simulink model "atrias"  (R2014a)
settings: Solver=FixedStepDiscrete  StartTime=0.0  StopTime=inf  FixedStep=0.001  RelTol=1e-3
libraries: xpcethercatlib x57, simulink x8, slrtlib x7
settings Model: xpc_rtwmakecfg_data=_xpcethercatlib_  SimulationMode=external  BufferReuse=off  Creator=drl  LastModifiedBy=drl
settings SolverCC: EnableConcurrentExecution=on  ConcurrentTasks=on
settings OptimizationCC: BlockReduction=off  OptimizeBlockIOStorage=off  BufferReuse=off  GlobalBufferReuse=off  ExpressionFolding=off  LocalBlockOutputs=off
settings HardwareCC: ProdIntDivRoundTo=Zero  ProdEndianess=LittleEndian  ProdHWDeviceType=Generic->32-bit x86 compatible
settings RTWCC: SystemTargetFile=slrt.tlc  TemplateMakefile=slrt_default_tmf  Description=Simulink Real-Time  ProcessScript=slrt_make_rtw_hook  RTWCompilerOptimization=On
settings SimulinkRealTimeCC: GeneratePreprocessorConditionals=Disable all  EnableShiftOperators=on

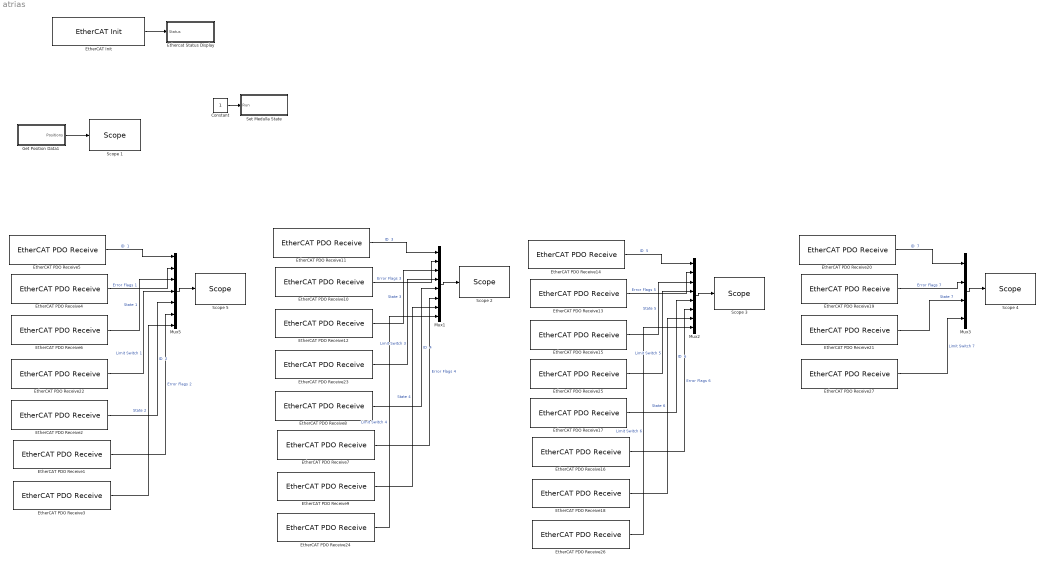
== system atrias ==
  Constant : Constant
  "EtherCAT Init " : xpcethercatlib/EtherCAT Init   Priority=0  config_file=C:\Users\drl\Documents\MATLAB\eni_atrias.xml  device_id=0  pci_bus=4  pci_slot=0  enaDebug=off  enaDC=on  errLink=off  masterDbg=off  stateChgDbg=off  baseClock=off  masterCfg=off  logFile='c:\dbglog.txt'  sample_time=0.001000
  EtherCAT PDO Receive1 : xpcethercatlib/EtherCAT PDO Receive  Priority=2  sig_name=Box 2 (ATRIAS 2.1 Boom (Medulla 1.5)).uController Status.Error Flags  sig_offset=992  sig_type=uint8  type_size=8  sig_dim=1  device_id=0  sample_time=0.001000
  EtherCAT PDO Receive10 : xpcethercatlib/EtherCAT PDO Receive  Priority=2  sig_name=Box 3 (ATRIAS 2.1 Hip (Medulla 1.5)).uController Status.Error Flags  sig_offset=1184  sig_type=uint8  type_size=8  sig_dim=1  device_id=0  sample_time=0.001000
  EtherCAT PDO Receive11 : xpcethercatlib/EtherCAT PDO Receive  Priority=2  sig_name=Box 3 (ATRIAS 2.1 Hip (Medulla 1.5)).uController Status.ID  sig_offset=1160  sig_type=uint8  type_size=8  sig_dim=1  device_id=0  sample_time=0.001000
  EtherCAT PDO Receive12 : xpcethercatlib/EtherCAT PDO Receive  Priority=2  sig_name=Box 3 (ATRIAS 2.1 Hip (Medulla 1.5)).uController Status.State  sig_offset=1168  sig_type=uint8  type_size=8  sig_dim=1  device_id=0  sample_time=0.001000
  EtherCAT PDO Receive13 : xpcethercatlib/EtherCAT PDO Receive  Priority=2  sig_name=Box 5 (ATRIAS 2.1 Leg (Medulla 1.5)).uController Status.Error Flags  sig_offset=1808  sig_type=uint8  type_size=8  sig_dim=1  device_id=0  sample_time=0.001000
  EtherCAT PDO Receive14 : xpcethercatlib/EtherCAT PDO Receive  Priority=2  sig_name=Box 5 (ATRIAS 2.1 Leg (Medulla 1.5)).uController Status.ID  sig_offset=1784  sig_type=uint8  type_size=8  sig_dim=1  device_id=0  sample_time=0.001000
  EtherCAT PDO Receive15 : xpcethercatlib/EtherCAT PDO Receive  Priority=2  sig_name=Box 5 (ATRIAS 2.1 Leg (Medulla 1.5)).uController Status.State  sig_offset=1792  sig_type=uint8  type_size=8  sig_dim=1  device_id=0  sample_time=0.001000
  EtherCAT PDO Receive16 : xpcethercatlib/EtherCAT PDO Receive  Priority=2  sig_name=Box 6 (ATRIAS 2.1 Leg (Medulla 1.5)).uController Status.Error Flags  sig_offset=2184  sig_type=uint8  type_size=8  sig_dim=1  device_id=0  sample_time=0.001000
  EtherCAT PDO Receive17 : xpcethercatlib/EtherCAT PDO Receive  Priority=2  sig_name=Box 6 (ATRIAS 2.1 Leg (Medulla 1.5)).uController Status.ID  sig_offset=2160  sig_type=uint8  type_size=8  sig_dim=1  device_id=0  sample_time=0.001000
  EtherCAT PDO Receive18 : xpcethercatlib/EtherCAT PDO Receive  Priority=2  sig_name=Box 6 (ATRIAS 2.1 Leg (Medulla 1.5)).uController Status.State  sig_offset=2168  sig_type=uint8  type_size=8  sig_dim=1  device_id=0  sample_time=0.001000
  EtherCAT PDO Receive19 : xpcethercatlib/EtherCAT PDO Receive  Priority=2  sig_name=Box 7 (ATRIAS 2.1 Hip (Medulla 1.5)).uController Status.Error Flags  sig_offset=2560  sig_type=uint8  type_size=8  sig_dim=1  device_id=0  sample_time=0.001000
  EtherCAT PDO Receive2 : xpcethercatlib/EtherCAT PDO Receive  Priority=2  sig_name=Box 2 (ATRIAS 2.1 Boom (Medulla 1.5)).uController Status.ID  sig_offset=968  sig_type=uint8  type_size=8  sig_dim=1  device_id=0  sample_time=0.001000
  EtherCAT PDO Receive20 : xpcethercatlib/EtherCAT PDO Receive  Priority=2  sig_name=Box 7 (ATRIAS 2.1 Hip (Medulla 1.5)).uController Status.ID  sig_offset=2536  sig_type=uint8  type_size=8  sig_dim=1  device_id=0  sample_time=0.001000
  EtherCAT PDO Receive21 : xpcethercatlib/EtherCAT PDO Receive  Priority=2  sig_name=Box 7 (ATRIAS 2.1 Hip (Medulla 1.5)).uController Status.State  sig_offset=2544  sig_type=uint8  type_size=8  sig_dim=1  device_id=0  sample_time=0.001000
  EtherCAT PDO Receive22 : xpcethercatlib/EtherCAT PDO Receive  Priority=2  sig_name=Box 1 (ATRIAS 2.1 Leg (Medulla 1.5)).uController Status.Limit Switch  sig_offset=624  sig_type=uint8  type_size=8  sig_dim=1  device_id=0  sample_time=0.001000
  EtherCAT PDO Receive23 : xpcethercatlib/EtherCAT PDO Receive  Priority=2  sig_name=Box 3 (ATRIAS 2.1 Hip (Medulla 1.5)).uController Status.Limit Switch  sig_offset=1192  sig_type=uint8  type_size=8  sig_dim=1  device_id=0  sample_time=0.001000
  EtherCAT PDO Receive24 : xpcethercatlib/EtherCAT PDO Receive  Priority=2  sig_name=Box 4 (ATRIAS 2.1 Leg (Medulla 1.5)).uController Status.Limit Switch  sig_offset=1440  sig_type=uint8  type_size=8  sig_dim=1  device_id=0  sample_time=0.001000
  EtherCAT PDO Receive25 : xpcethercatlib/EtherCAT PDO Receive  Priority=2  sig_name=Box 5 (ATRIAS 2.1 Leg (Medulla 1.5)).uController Status.Limit Switch  sig_offset=1816  sig_type=uint8  type_size=8  sig_dim=1  device_id=0  sample_time=0.001000
  EtherCAT PDO Receive26 : xpcethercatlib/EtherCAT PDO Receive  Priority=2  sig_name=Box 6 (ATRIAS 2.1 Leg (Medulla 1.5)).uController Status.State  sig_offset=2168  sig_type=uint8  type_size=8  sig_dim=1  device_id=0  sample_time=0.001000
  EtherCAT PDO Receive27 : xpcethercatlib/EtherCAT PDO Receive  Priority=2  sig_name=Box 7 (ATRIAS 2.1 Hip (Medulla 1.5)).uController Status.Limit Switch  sig_offset=2568  sig_type=uint8  type_size=8  sig_dim=1  device_id=0  sample_time=0.001000
  EtherCAT PDO Receive3 : xpcethercatlib/EtherCAT PDO Receive  Priority=2  sig_name=Box 2 (ATRIAS 2.1 Boom (Medulla 1.5)).uController Status.State  sig_offset=976  sig_type=uint8  type_size=8  sig_dim=1  device_id=0  sample_time=0.001000
  EtherCAT PDO Receive4 : xpcethercatlib/EtherCAT PDO Receive  Priority=2  sig_name=Box 1 (ATRIAS 2.1 Leg (Medulla 1.5)).uController Status.Error Flags  sig_offset=616  sig_type=uint8  type_size=8  sig_dim=1  device_id=0  sample_time=0.001000
  EtherCAT PDO Receive5 : xpcethercatlib/EtherCAT PDO Receive  Priority=2  sig_name=Box 1 (ATRIAS 2.1 Leg (Medulla 1.5)).uController Status.ID  sig_offset=592  sig_type=uint8  type_size=8  sig_dim=1  device_id=0  sample_time=0.001000
  EtherCAT PDO Receive6 : xpcethercatlib/EtherCAT PDO Receive  Priority=2  sig_name=Box 1 (ATRIAS 2.1 Leg (Medulla 1.5)).uController Status.State  sig_offset=600  sig_type=uint8  type_size=8  sig_dim=1  device_id=0  sample_time=0.001000
  EtherCAT PDO Receive7 : xpcethercatlib/EtherCAT PDO Receive  Priority=2  sig_name=Box 4 (ATRIAS 2.1 Leg (Medulla 1.5)).uController Status.Error Flags  sig_offset=1432  sig_type=uint8  type_size=8  sig_dim=1  device_id=0  sample_time=0.001000
  EtherCAT PDO Receive8 : xpcethercatlib/EtherCAT PDO Receive  Priority=2  sig_name=Box 4 (ATRIAS 2.1 Leg (Medulla 1.5)).uController Status.ID  sig_offset=1408  sig_type=uint8  type_size=8  sig_dim=1  device_id=0  sample_time=0.001000
  EtherCAT PDO Receive9 : xpcethercatlib/EtherCAT PDO Receive  Priority=2  sig_name=Box 4 (ATRIAS 2.1 Leg (Medulla 1.5)).uController Status.State  sig_offset=1416  sig_type=uint8  type_size=8  sig_dim=1  device_id=0  sample_time=0.001000
  Ethercat Status Display : Subsystem
  Get Position Data1 : Subsystem
  Mux1 : Mux  Inputs=8
  Mux2 : Mux  Inputs=8
  Mux3 : Mux
  Mux5 : Mux  Inputs=7
  Scope 1 : slrtlib/Displays and Logging/Scope   scopeno=1  scopetype=Target  autostart=on  viewmode=Numerical  formatstr='%15.6f'  grid=on  ylimits=[0,0]  nosamples=100  noprepostsamples=0  interleave=1  triggermode=FreeRun  triggersignal=1  trigsignalfromport=off  triggerlevel=0.0  triggerslope=Either  triggerscope=1  triggersample=0  filename=data.dat  mode=Lazy  writesize=512  autorestart=off  dynamicfilemode=off  maxwritefilesize=512*1024^2
  Scope 2 : slrtlib/Displays and Logging/Scope   scopeno=4  scopetype=Target  autostart=on  viewmode=Numerical  formatstr='%15.6f'  grid=on  ylimits=[0,0]  nosamples=100  noprepostsamples=0  interleave=1  triggermode=FreeRun  triggersignal=1  trigsignalfromport=off  triggerlevel=0.0  triggerslope=Either  triggerscope=1  triggersample=0  filename=data.dat  mode=Lazy  writesize=512  autorestart=off  dynamicfilemode=off  maxwritefilesize=512*1024^2
  Scope 3 : slrtlib/Displays and Logging/Scope   scopeno=5  scopetype=Target  autostart=on  viewmode=Numerical  formatstr='%15.6f'  grid=on  ylimits=[0,0]  nosamples=100  noprepostsamples=0  interleave=1  triggermode=FreeRun  triggersignal=1  trigsignalfromport=off  triggerlevel=0.0  triggerslope=Either  triggerscope=1  triggersample=0  filename=data.dat  mode=Lazy  writesize=512  autorestart=off  dynamicfilemode=off  maxwritefilesize=512*1024^2
  Scope 4 : slrtlib/Displays and Logging/Scope   scopeno=7  scopetype=Target  autostart=on  viewmode=Numerical  formatstr='%15.6f'  grid=on  ylimits=[0,0]  nosamples=100  noprepostsamples=0  interleave=1  triggermode=FreeRun  triggersignal=1  trigsignalfromport=off  triggerlevel=0.0  triggerslope=Either  triggerscope=1  triggersample=0  filename=data.dat  mode=Lazy  writesize=512  autorestart=off  dynamicfilemode=off  maxwritefilesize=512*1024^2
  Scope 5 : slrtlib/Displays and Logging/Scope   scopeno=3  scopetype=Target  autostart=on  viewmode=Numerical  formatstr='%15.6f'  grid=on  ylimits=[0,0]  nosamples=100  noprepostsamples=0  interleave=1  triggermode=FreeRun  triggersignal=1  trigsignalfromport=off  triggerlevel=0.0  triggerslope=Either  triggerscope=1  triggersample=0  filename=data.dat  mode=Lazy  writesize=512  autorestart=off  dynamicfilemode=off  maxwritefilesize=512*1024^2
  Set Medulla State : Subsystem
  wires:
  "EtherCAT Init "/1 -> Ethercat Status Display/1(Status)
  Mux5/1 -> Scope 5/1
  EtherCAT PDO Receive5/1 -> Mux5/1  "ID  1"
  EtherCAT PDO Receive4/1 -> Mux5/2  "Error Flags 1"
  EtherCAT PDO Receive6/1 -> Mux5/3  "State 1"
  EtherCAT PDO Receive2/1 -> Mux5/5  "ID  2"
  EtherCAT PDO Receive1/1 -> Mux5/6  "Error Flags 2"
  EtherCAT PDO Receive3/1 -> Mux5/7  "State 2"
  Mux1/1 -> Scope 2/1
  EtherCAT PDO Receive11/1 -> Mux1/1  "ID  3"
  EtherCAT PDO Receive10/1 -> Mux1/2  "Error Flags 3"
  EtherCAT PDO Receive12/1 -> Mux1/3  "State 3"
  EtherCAT PDO Receive8/1 -> Mux1/5  "ID  4"
  EtherCAT PDO Receive7/1 -> Mux1/6  "Error Flags 4"
  EtherCAT PDO Receive9/1 -> Mux1/7  "State 4"
  Mux2/1 -> Scope 3/1
  EtherCAT PDO Receive14/1 -> Mux2/1  "ID  5"
  EtherCAT PDO Receive13/1 -> Mux2/2  "Error Flags 5"
  EtherCAT PDO Receive15/1 -> Mux2/3  "State 5"
  EtherCAT PDO Receive17/1 -> Mux2/5  "ID  6"
  EtherCAT PDO Receive16/1 -> Mux2/6  "Error Flags 6"
  EtherCAT PDO Receive18/1 -> Mux2/7  "State 6"
  Mux3/1 -> Scope 4/1
  EtherCAT PDO Receive20/1 -> Mux3/1  "ID  7"
  EtherCAT PDO Receive19/1 -> Mux3/2  "Error Flags 7"
  EtherCAT PDO Receive21/1 -> Mux3/3  "State 7"
  EtherCAT PDO Receive22/1 -> Mux5/4  "Limit Switch 1"
  EtherCAT PDO Receive23/1 -> Mux1/4  "Limit Switch 3"
  EtherCAT PDO Receive24/1 -> Mux1/8  "Limit Switch 4"
  EtherCAT PDO Receive25/1 -> Mux2/4  "Limit Switch 5"
  EtherCAT PDO Receive26/1 -> Mux2/8  "Limit Switch 6"
  EtherCAT PDO Receive27/1 -> Mux3/4  "Limit Switch 7"
  Get Position Data1/1("Positions ") -> Scope 1/1
  Constant/1 -> Set Medulla State/1(Run)

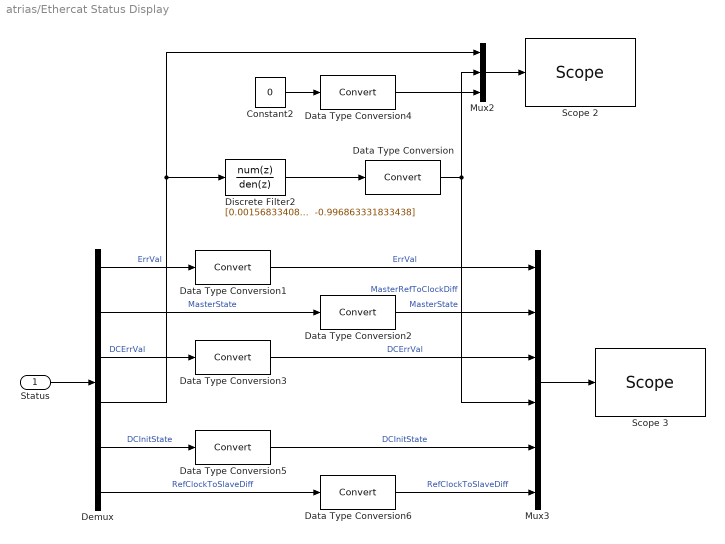
== system atrias/Ethercat Status Display ==
  Status : Inport
  Constant2 : Constant  Value=0  OutDataTypeStr=Inherit: Inherit via back propagation  SampleTime=-1
  Data Type Conversion{,1..6} (7 alike) : DataTypeConversion
  Demux : Demux  Outputs=6
  Discrete Filter2 : DiscreteFilter  Numerator="[0.001568334083281   0.001568334083281]"  Denominator="[1.000000000000000  -0.996863331833438]"  a0EqualsOne=on
  Mux2 : Mux  Inputs=3
  Mux3 : Mux  Inputs=6
  Scope 2 : slrtlib/Displays and Logging/Scope   scopeno=6  scopetype=Target  autostart=on  viewmode=Graphical rolling  formatstr='%f'  grid=on  ylimits=[0,0]  nosamples=10000  noprepostsamples=0  interleave=1  triggermode=FreeRun  triggersignal=1  trigsignalfromport=off  triggerlevel=0.0  triggerslope=Either  triggerscope=1  triggersample=0  filename=data.dat  mode=Lazy  writesize=512  autorestart=off  dynamicfilemode=off  maxwritefilesize=512*1024^2
  Scope 3 : slrtlib/Displays and Logging/Scope   scopeno=2  scopetype=Target  autostart=on  viewmode=Numerical  formatstr='%15.6f'  grid=on  ylimits=[0,0]  nosamples=100  noprepostsamples=0  interleave=1  triggermode=FreeRun  triggersignal=1  trigsignalfromport=off  triggerlevel=0.0  triggerslope=Either  triggerscope=1  triggersample=0  filename=data.dat  mode=Lazy  writesize=512  autorestart=off  dynamicfilemode=off  maxwritefilesize=512*1024^2
  wires:
  Status/1 -> Demux/1
  Demux/4 -> Discrete Filter2/1, Mux2/1
  Discrete Filter2/1 -> Data Type Conversion/1
  Mux2/1 -> Scope 2/1
  Constant2/1 -> Data Type Conversion4/1
  Data Type Conversion4/1 -> Mux2/3
  Mux3/1 -> Scope 3/1
  Data Type Conversion/1 -> Mux3/4, Mux2/2  "MasterRefToClockDiff"
  Data Type Conversion1/1 -> Mux3/1  "ErrVal"
  Data Type Conversion2/1 -> Mux3/2  "MasterState"
  Data Type Conversion3/1 -> Mux3/3  "DCErrVal"
  Data Type Conversion5/1 -> Mux3/5  "DCInitState"
  Data Type Conversion6/1 -> Mux3/6  "RefClockToSlaveDiff"
  Demux/1 -> Data Type Conversion1/1  "ErrVal"
  Demux/2 -> Data Type Conversion2/1  "MasterState"
  Demux/3 -> Data Type Conversion3/1  "DCErrVal"
  Demux/5 -> Data Type Conversion5/1  "DCInitState"
  Demux/6 -> Data Type Conversion6/1  "RefClockToSlaveDiff"

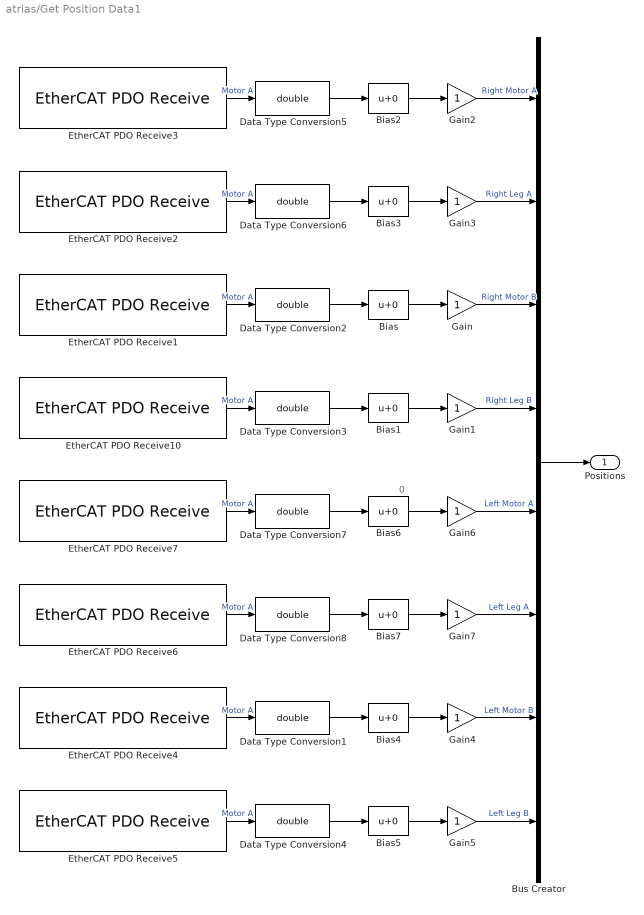
== system atrias/Get Position Data1 ==
  note: 0
  Bias{,1..7} (8 alike) : Bias
  Bus Creator : BusCreator  Inputs=8
  Data Type Conversion{1..8} (8 alike) : DataTypeConversion  OutDataTypeStr=double
  EtherCAT PDO Receive{1,3..4,7} (4 alike) : xpcethercatlib/EtherCAT PDO Receive  Priority=2  sig_name=Box 1 (ATRIAS 2.1 Leg (Medulla 1.5)).Motor Encoder.Motor Encoder  sig_offset=648  sig_type=uint32  type_size=32  sig_dim=1  device_id=0  sample_time=0.001000
  EtherCAT PDO Receive{2,5..6,10} (4 alike) : xpcethercatlib/EtherCAT PDO Receive  Priority=2  sig_name=Box 1 (ATRIAS 2.1 Leg (Medulla 1.5)).Leg Encoder.Leg Encoder  sig_offset=696  sig_type=uint32  type_size=32  sig_dim=1  device_id=0  sample_time=0.001000
  Gain{,1..7} (8 alike) : Gain
  "Positions " : Outport
  wires:
  Gain/1 -> Bus Creator/3  "Right Motor B"
  Gain1/1 -> Bus Creator/4  "Right Leg B"
  Gain2/1 -> Bus Creator/1  "Right Motor A"
  Gain3/1 -> Bus Creator/2  "Right Leg A"
  EtherCAT PDO Receive1/1 -> Data Type Conversion2/1  "Motor A"
  Data Type Conversion2/1 -> Bias/1
  Bias/1 -> Gain/1
  EtherCAT PDO Receive10/1 -> Data Type Conversion3/1  "Motor A"
  Data Type Conversion3/1 -> Bias1/1
  Bias1/1 -> Gain1/1
  EtherCAT PDO Receive3/1 -> Data Type Conversion5/1  "Motor A"
  Data Type Conversion5/1 -> Bias2/1
  Bias2/1 -> Gain2/1
  EtherCAT PDO Receive2/1 -> Data Type Conversion6/1  "Motor A"
  Data Type Conversion6/1 -> Bias3/1
  Bias3/1 -> Gain3/1
  Bus Creator/1 -> "Positions "/1
  Gain4/1 -> Bus Creator/7  "Left Motor B"
  Gain5/1 -> Bus Creator/8  "Left Leg B"
  Gain6/1 -> Bus Creator/5  "Left Motor A"
  Gain7/1 -> Bus Creator/6  "Left Leg A"
  EtherCAT PDO Receive4/1 -> Data Type Conversion1/1  "Motor A"
  Data Type Conversion1/1 -> Bias4/1
  Bias4/1 -> Gain4/1
  EtherCAT PDO Receive5/1 -> Data Type Conversion4/1  "Motor A"
  Data Type Conversion4/1 -> Bias5/1
  Bias5/1 -> Gain5/1
  EtherCAT PDO Receive7/1 -> Data Type Conversion7/1  "Motor A"
  Data Type Conversion7/1 -> Bias6/1
  Bias6/1 -> Gain6/1
  EtherCAT PDO Receive6/1 -> Data Type Conversion8/1  "Motor A"
  Data Type Conversion8/1 -> Bias7/1
  Bias7/1 -> Gain7/1

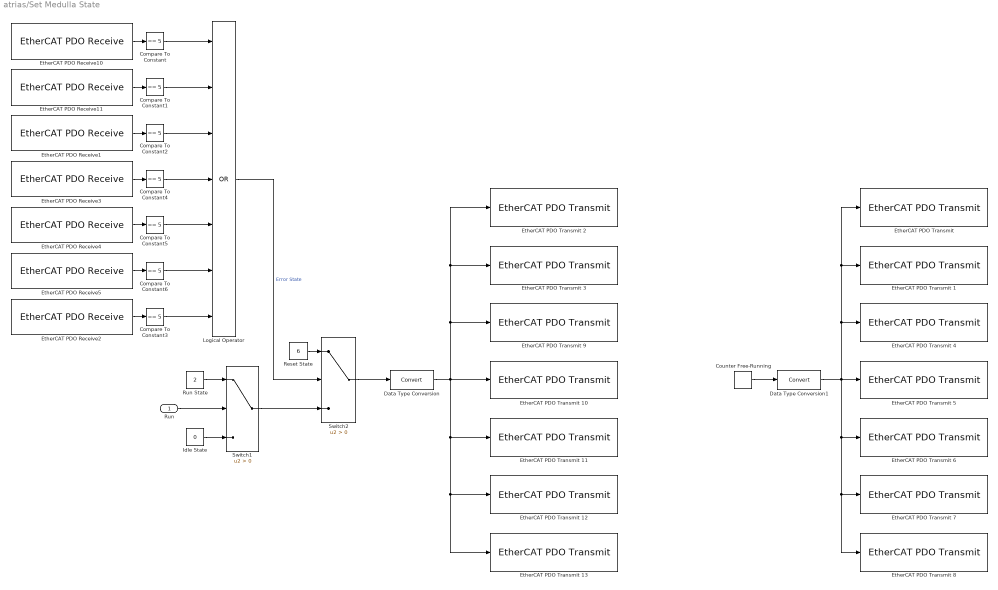
== system atrias/Set Medulla State ==
  Run : Inport
  Compare To Constant{,1..6} (7 alike) : simulink/Logic and Bit Operations/Compare To Constant  relop===  const=5  OutDataTypeStr=boolean
  Counter Free-Running : simulink/Sources/Counter Free-Running  NumBits=16  tsamp=-1
  Data Type Conversion : DataTypeConversion
  Data Type Conversion1 : DataTypeConversion
  EtherCAT PDO Receive1 : xpcethercatlib/EtherCAT PDO Receive  Priority=2  sig_name=Box 3 (ATRIAS 2.1 Hip (Medulla 1.5)).uController Status.State  sig_offset=1168  sig_type=uint8  type_size=8  sig_dim=1  device_id=0  sample_time=0.001
  EtherCAT PDO Receive10 : xpcethercatlib/EtherCAT PDO Receive  Priority=2  sig_name=Box 1 (ATRIAS 2.1 Leg (Medulla 1.5)).uController Status.State  sig_offset=600  sig_type=uint8  type_size=8  sig_dim=1  device_id=0  sample_time=0.001
  EtherCAT PDO Receive11 : xpcethercatlib/EtherCAT PDO Receive  Priority=2  sig_name=Box 2 (ATRIAS 2.1 Boom (Medulla 1.5)).uController Status.State  sig_offset=976  sig_type=uint8  type_size=8  sig_dim=1  device_id=0  sample_time=0.001
  EtherCAT PDO Receive2 : xpcethercatlib/EtherCAT PDO Receive  Priority=2  sig_name=Box 7 (ATRIAS 2.1 Hip (Medulla 1.5)).uController Status.State  sig_offset=2544  sig_type=uint8  type_size=8  sig_dim=1  device_id=0  sample_time=0.001
  EtherCAT PDO Receive3 : xpcethercatlib/EtherCAT PDO Receive  Priority=2  sig_name=Box 4 (ATRIAS 2.1 Leg (Medulla 1.5)).uController Status.State  sig_offset=1416  sig_type=uint8  type_size=8  sig_dim=1  device_id=0  sample_time=0.001
  EtherCAT PDO Receive4 : xpcethercatlib/EtherCAT PDO Receive  Priority=2  sig_name=Box 5 (ATRIAS 2.1 Leg (Medulla 1.5)).uController Status.State  sig_offset=1792  sig_type=uint8  type_size=8  sig_dim=1  device_id=0  sample_time=0.001
  EtherCAT PDO Receive5 : xpcethercatlib/EtherCAT PDO Receive  Priority=2  sig_name=Box 6 (ATRIAS 2.1 Leg (Medulla 1.5)).uController Status.State  sig_offset=2168  sig_type=uint8  type_size=8  sig_dim=1  device_id=0  sample_time=0.001
  "EtherCAT PDO Transmit " : xpcethercatlib/EtherCAT PDO Transmit   Priority=3  sig_name=Box 1 (ATRIAS 2.1 Leg (Medulla 1.5)).uControllerInput.Counter  sig_offset=600  sig_type=uint16  type_size=16  sig_dim=1  device_id=0  sample_time=0.001
  EtherCAT PDO Transmit 1 : xpcethercatlib/EtherCAT PDO Transmit   Priority=3  sig_name=Box 2 (ATRIAS 2.1 Boom (Medulla 1.5)).uControllerInput.Counter  sig_offset=976  sig_type=uint16  type_size=16  sig_dim=1  device_id=0  sample_time=0.001
  EtherCAT PDO Transmit 10 : xpcethercatlib/EtherCAT PDO Transmit   Priority=3  sig_name=Box 4 (ATRIAS 2.1 Leg (Medulla 1.5)).uControllerInput.Command  sig_offset=1408  sig_type=uint8  type_size=8  sig_dim=1  device_id=0  sample_time=0.001
  EtherCAT PDO Transmit 11 : xpcethercatlib/EtherCAT PDO Transmit   Priority=3  sig_name=Box 5 (ATRIAS 2.1 Leg (Medulla 1.5)).uControllerInput.Command  sig_offset=1784  sig_type=uint8  type_size=8  sig_dim=1  device_id=0  sample_time=0.001
  EtherCAT PDO Transmit 12 : xpcethercatlib/EtherCAT PDO Transmit   Priority=3  sig_name=Box 6 (ATRIAS 2.1 Leg (Medulla 1.5)).uControllerInput.Command  sig_offset=2160  sig_type=uint8  type_size=8  sig_dim=1  device_id=0  sample_time=0.001
  EtherCAT PDO Transmit 13 : xpcethercatlib/EtherCAT PDO Transmit   Priority=3  sig_name=Box 7 (ATRIAS 2.1 Hip (Medulla 1.5)).uControllerInput.Command  sig_offset=2536  sig_type=uint8  type_size=8  sig_dim=1  device_id=0  sample_time=0.001
  EtherCAT PDO Transmit 2 : xpcethercatlib/EtherCAT PDO Transmit   Priority=3  sig_name=Box 1 (ATRIAS 2.1 Leg (Medulla 1.5)).uControllerInput.Command  sig_offset=592  sig_type=uint8  type_size=8  sig_dim=1  device_id=0  sample_time=0.001
  EtherCAT PDO Transmit 3 : xpcethercatlib/EtherCAT PDO Transmit   Priority=3  sig_name=Box 2 (ATRIAS 2.1 Boom (Medulla 1.5)).uControllerInput.Command  sig_offset=968  sig_type=uint8  type_size=8  sig_dim=1  device_id=0  sample_time=0.001
  EtherCAT PDO Transmit 4 : xpcethercatlib/EtherCAT PDO Transmit   Priority=3  sig_name=Box 3 (ATRIAS 2.1 Hip (Medulla 1.5)).uControllerInput.Counter  sig_offset=1168  sig_type=uint16  type_size=16  sig_dim=1  device_id=0  sample_time=0.001
  EtherCAT PDO Transmit 5 : xpcethercatlib/EtherCAT PDO Transmit   Priority=3  sig_name=Box 4 (ATRIAS 2.1 Leg (Medulla 1.5)).uControllerInput.Counter  sig_offset=1416  sig_type=uint16  type_size=16  sig_dim=1  device_id=0  sample_time=0.001
  EtherCAT PDO Transmit 6 : xpcethercatlib/EtherCAT PDO Transmit   Priority=3  sig_name=Box 5 (ATRIAS 2.1 Leg (Medulla 1.5)).uControllerInput.Counter  sig_offset=1792  sig_type=uint16  type_size=16  sig_dim=1  device_id=0  sample_time=0.001
  EtherCAT PDO Transmit 7 : xpcethercatlib/EtherCAT PDO Transmit   Priority=3  sig_name=Box 6 (ATRIAS 2.1 Leg (Medulla 1.5)).uControllerInput.Counter  sig_offset=2168  sig_type=uint16  type_size=16  sig_dim=1  device_id=0  sample_time=0.001
  EtherCAT PDO Transmit 8 : xpcethercatlib/EtherCAT PDO Transmit   Priority=3  sig_name=Box 7 (ATRIAS 2.1 Hip (Medulla 1.5)).uControllerInput.Counter  sig_offset=2544  sig_type=uint16  type_size=16  sig_dim=1  device_id=0  sample_time=0.001
  EtherCAT PDO Transmit 9 : xpcethercatlib/EtherCAT PDO Transmit   Priority=3  sig_name=Box 3 (ATRIAS 2.1 Hip (Medulla 1.5)).uControllerInput.Command  sig_offset=1160  sig_type=uint8  type_size=8  sig_dim=1  device_id=0  sample_time=0.001
  Idle State : Constant  Value=0
  Logical Operator : Logic  Operator=OR  Inputs=7  AllPortsSameDT=off  OutDataTypeStr=boolean
  Reset State : Constant  Value=6
  Run State : Constant  Value=2
  Switch1 : Switch  Criteria=u2 > Threshold
  Switch2 : Switch  Criteria=u2 > Threshold
  wires:
  Data Type Conversion1/1 -> EtherCAT PDO Transmit 8/1, EtherCAT PDO Transmit 7/1, EtherCAT PDO Transmit 6/1, EtherCAT PDO Transmit 5/1, EtherCAT PDO Transmit 4/1, "EtherCAT PDO Transmit "/1, EtherCAT PDO Transmit 1/1
  Counter Free-Running/1 -> Data Type Conversion1/1
  Run/1 -> Switch1/2
  Run State/1 -> Switch1/1
  Idle State/1 -> Switch1/3
  Compare To Constant1/1 -> Logical Operator/2
  Compare To Constant/1 -> Logical Operator/1
  EtherCAT PDO Receive10/1 -> Compare To Constant/1
  EtherCAT PDO Receive11/1 -> Compare To Constant1/1
  Logical Operator/1 -> Switch2/2  "Error State"
  Switch1/1 -> Switch2/3
  Reset State/1 -> Switch2/1
  Switch2/1 -> Data Type Conversion/1
  Data Type Conversion/1 -> EtherCAT PDO Transmit 13/1, EtherCAT PDO Transmit 12/1, EtherCAT PDO Transmit 11/1, EtherCAT PDO Transmit 10/1, EtherCAT PDO Transmit 9/1, EtherCAT PDO Transmit 2/1, EtherCAT PDO Transmit 3/1
  EtherCAT PDO Receive1/1 -> Compare To Constant2/1
  Compare To Constant2/1 -> Logical Operator/3
  EtherCAT PDO Receive3/1 -> Compare To Constant4/1
  Compare To Constant4/1 -> Logical Operator/4
  EtherCAT PDO Receive4/1 -> Compare To Constant5/1
  Compare To Constant5/1 -> Logical Operator/5
  EtherCAT PDO Receive5/1 -> Compare To Constant6/1
  Compare To Constant6/1 -> Logical Operator/6
  EtherCAT PDO Receive2/1 -> Compare To Constant3/1
  Compare To Constant3/1 -> Logical Operator/7
